simulink model "synchronverter_simulation"  (R2023a)
settings: Solver=ode23tb  StartTime=0.0  StopTime=9  FixedStep=1e-5  MaxStep=0.2e-3  RelTol=1e-3
model workspace (MAT data in the model file):
  Dp = 0.2026
  Dq = 117.88
  Ki = 9
  Kp = 1
  L = 0.0002
  Lg = 0.00015
  Ls = 0.00045
  Pset = 80
  Qset = 60
  R = 0.05
  Rg = 0.045
  Rs = 0.135
  Vdclink = 42
  Vlgrms = 380
  Vnpeak = 16.9667989517
  Wn = 314.159265359
  Ws = 94247.7796077
  fg = 50
  fs = 15000
  tf = 0.002
  tv = 0.02
libraries: simulink_extras x5, spsThreePhaseVIMeasurementLib x5, spsThreePhaseBreakerLib x4, spsPower3phInstantaneousLib x4, cstblocks x3, spsGroundLib x3, spsThreePhaseParallelRLCLoadLib x2, spsThreePhaseSeriesRLCBranchLib x2, spsDCVoltageSourceLib x2, spsThreePhaseProgrammableVoltageSourceLib x1, spsThreePhaseParallelRLCBranchLib x1, slpidlib x1
settings Model: Creator=Hi  LastModifiedBy=Aminsystem
settings SolverCC: AlgebraicLoopSolver=TrustRegion
settings DataIOCC: ReturnWorkspaceOutputs=off
settings DebuggingCC: AlgebraicLoopMsg=none  ArithmeticOperatorsInVariantConditions=warning
settings ModelReferenceCC: EnableRefExpFcnMdlSchedulingChecks=on
settings SFSimCC: SimUseLocalCustomCode=off  CustomCodeUndefinedFunction=UseInterfaceOnly
settings RTWCC: RTWUseLocalCustomCode=off
settings ConfigComp: DVTestSuiteOptimization=CombinedObjectives (Nonlinear Extended)

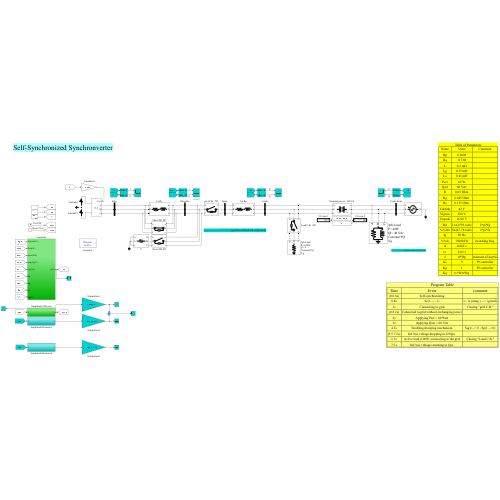
[thumbnail: Simulink's stored preview of the top-level diagram]
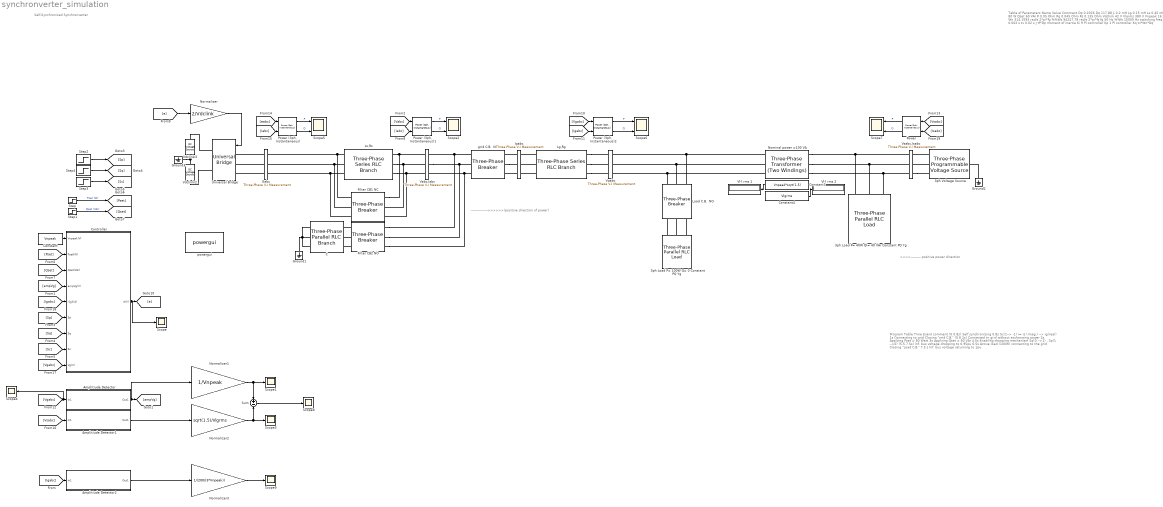
== system synchronverter_simulation ==
  note: <<<<---------- positive power direction
  note: ----------------->>>>>>(positive direction of power)
  note: Table of Parameters
      | Name
      | Value
      | Comment
      |
      | Dp
      | 0.2026
      |
      | Dq
      | 117.88
      |
      | L
      | 0.2 mH
      |
      | Lg
      | 0.15 mH
      |
      | Ls
      | 0.45 mH
      |
      | Pset
      | 80 W
      |
      | Qset
      | 60 VAr
      |
      | R
      | 0.05 Ohm
      |
      | Rg
      | 0.045 Ohm
      |
      | Rs
      | 0.135 Ohm
      |
      | Vdclink
      | 42 V
      |
      | Vlgrms
      | 380 V
      |
      | Vnpeak
      | 16.96 V
      |
      | Wn
      | 314.1593 rad/s
      | 2*pi*fg
      |
      | %%Ws
      | 94247.78 rad/s
      | 2*pi*fs
      |
      | fg
      | 50 Hz
      |
      | %%fs
      | 15000 Hz
      | switching freq.
      |
      | tf
      | 0.002 s
      |
      | tv
      | 0.02 s
      |
      | J
      | tf*Dp
      | moment of inertia
      |
      | Ki
      | 9
      | PI controller
      |
      | Kp
      | 1
      | PI controller
      |
      | Kq
      | tv*Wn*Dq
  note: Program Table
      | Time
      | Event
      | comment
      |
      | (0 0.8s)
      | Self synchronizing
      |
      | 0.8s
      | Sc(1--> -1)
      | i= is (imag.) --> ig(real)
      |
      | 1s
      | Connecting to grid
      | Closing "grid C.B."
      |
      | (0.8 2s)
      | Connected to grid without exchanging power
      |
      | 2s
      | Applying Pset = 80 Watt
      |
      | 3s
      | Applying Qset = 60 VAr
      |
      | 4.5s
      | Enabling drooping mechanism
      | Sq(0 -->1) , Sp(1 -->0)
      |
      | (5.5 7.5s)
      | Inf. bus voltage dropping to 0.95pu
      |
      | 6.5s
      | Active load (100W) connecting to the grid
      | Closing "Load C.B."
      |
      | 7.5 s
      | Inf. bus voltage returning to 1pu
  note: Self-Synchronized Synchronverter
  3ph Voltage Source : spsThreePhaseProgrammableVoltageSourceLib/Three-Phase Programmable Voltage Source  PositiveSequence=[Vlgrms 0 fg]  VariationEntity=Amplitude  VariationType=Table of time-amplitude pairs  VariationTypeAlt=Step  VariationStep=0.5  VariationRate=10  VariationMagnitude=0.3  VariationFrequency=2  VariationTiming=[1 2]  VariationPhaseA=off  Amplitudes=[1 0.95 1]  TimeValues=[0 5.5 7.5]  HarmonicGeneration=off  HarmonicA=[3 0.2 -25 0]  HarmonicB=[2 0.15 35 2]  Timing="[0.05  3]"  BusType=swing  Pref=0  Qref=0  Qmin=-inf  Qmax=inf
  3ph Load P= 100W Q= 0 Constant PQ Yg : spsThreePhaseParallelRLCLoadLib/Three-Phase Parallel RLC Load  LConnTagsString=A|B|C  Configuration=Y (grounded)  NominalVoltage=Vnpeak*sqrt(1.5)  Vabc=[1e3 1e3 1e3]  Vabcp=[1e3 1e3 1e3]  NominalFrequency=fg  UnbalancedPower=off  ActivePower=100  InductivePower=0  CapacitivePower=0  Pabc=[10e3 9e3 11e3]  QLabc=[100 90 110]  QCabc=[100 90 110]  Pabcp=[10e3 9e3 11e3]  QLabcp=[100 90 110]  QCabcp=[100 90 110]  Measurements=None  LoadType=constant PQ
  3ph Load P= 40W Ql= 40 VAr Constant PQ Yg : spsThreePhaseParallelRLCLoadLib/Three-Phase Parallel RLC Load  LConnTagsString=A|B|C  Configuration=Y (grounded)  NominalVoltage=Vlgrms  Vabc=[1e3 1e3 1e3]  Vabcp=[1e3 1e3 1e3]  NominalFrequency=fg  UnbalancedPower=off  ActivePower=40  InductivePower=40  CapacitivePower=0  Pabc=[10e3 9e3 11e3]  QLabc=[100 90 110]  QCabc=[100 90 110]  Pabcp=[10e3 9e3 11e3]  QLabcp=[100 90 110]  QCabcp=[100 90 110]  Measurements=None  LoadType=constant PQ
  Amplitiude Detector : Subsystem
  Amplitiude Detector1 : Subsystem
  Amplitiude Detector2 : Subsystem
  C : spsThreePhaseParallelRLCBranchLib/Three-Phase Parallel RLC Branch  LConnTagsString=A|B|C  RConnTagsString=A|B|C  BranchType=C  Resistance=inf  Inductance=1e3  Capacitance=1/(L*Wn*Ws)*1+(22e-6)*0  Measurements=None
  Constant : Constant  Value=Vnpeak
  Constant3 : Constant  Value=Vnpeak*sqrt(1.5)
  Constant4 : Constant  Value=Vlgrms
  Controller : Subsystem
  Eabc : spsThreePhaseVIMeasurementLib/Three-Phase V-I Measurement  VoltageMeasurement=phase-to-ground  SetLabelV=on  LabelV=eabc  Vpu=off  VpuLL=off  CurrentMeasurement=no  SetLabelI=on  LabelI=Iabc  Ipu=off  Pbase=100e6  Vbase=500e3  OutputType=Complex  PhasorSimulation=off  PSBequivalent=0
  Filter CB1 NC : spsThreePhaseBreakerLib/Three-Phase Breaker  InitialState=closed  SwitchA=on  SwitchB=on  SwitchC=on  SwitchTimes=[500]  External=off  BreakerResistance=0.01  SnubberResistance=1e7  SnubberCapacitance=inf  Measurements=None
  Filter CB2 NO : spsThreePhaseBreakerLib/Three-Phase Breaker  InitialState=open  SwitchA=on  SwitchB=on  SwitchC=on  SwitchTimes=[500]  External=off  BreakerResistance=0.01  SnubberResistance=1e7  SnubberCapacitance=inf  Measurements=None
  Ground1 : spsGroundLib/Ground  LConnTagsString=a
  Ground2 : spsGroundLib/Ground  LConnTagsString=a
  Ground3 : spsGroundLib/Ground  LConnTagsString=a
  Igabc : spsThreePhaseVIMeasurementLib/Three-Phase V-I Measurement  VoltageMeasurement=no  SetLabelV=off  LabelV=Vg3  Vpu=off  VpuLL=off  CurrentMeasurement=yes  SetLabelI=on  LabelI=Igabc  Ipu=off  Pbase=100e6  Vbase=500e3  OutputType=Complex  PhasorSimulation=off  PSBequivalent=0
  Lg,Rg : spsThreePhaseSeriesRLCBranchLib/Three-Phase Series RLC Branch  LConnTagsString=A|B|C  RConnTagsString=A|B|C  BranchType=RL  Resistance=Rg  Inductance=Lg  Capacitance=1e-6  Measurements=None
  Load C.B.  NO : spsThreePhaseBreakerLib/Three-Phase Breaker  InitialState=open  SwitchA=on  SwitchB=on  SwitchC=on  SwitchTimes=[6.5]  External=off  BreakerResistance=0.01  SnubberResistance=1e6  SnubberCapacitance=inf  Measurements=Breaker voltages
  Ls,Rs : spsThreePhaseSeriesRLCBranchLib/Three-Phase Series RLC Branch  LConnTagsString=A|B|C  RConnTagsString=A|B|C  BranchType=RL  Resistance=Rs  Inductance=Ls  Capacitance=1e-6  Measurements=None
  Nominal power =100 VA : spsThreePhaseTransformerTwoWindingsLib/Three-Phase Transformer (Two Windings)  Winding1Connection=Yg  Winding2Connection=Yg  CoreType=Three single-phase transformers  SetSaturation=off  Hysteresis=off  DataFile='hysteresis'  SetInitialFlux=off  Measurements=None  UNITS=pu  NominalPower=[ 100 , fg ]  Winding1=[ Vnpeak*sqrt(1.5) , 0.002 , 0.08 ]  Winding2=[Vlgrms , 0.002 , 0.08 ]  Rm=500  Lm=500  L0=0.5  Saturation=[ 0,0 ; 0.0024,1.2 ; 1.0,1.52 ]  InitialFluxes=[ 0.8 , -0.8 , 0.7 ]  BreakLoop=off  DiscreteSolver=Trapezoidal iterative  DataType=off  TransfoNumber=1
  Normalizer : Gain  Gain=2/Vdclink
  Normalizer1 : Gain  Gain=1/Vnpeak
  Normalizer2 : Gain  Gain=sqrt(1.5)/Vlgrms
  Normalizer3 : Gain  Gain=1/(200/(3*Vnpeak))
  Power : spsPower3phInstantaneousLib/Power (3ph, Instantaneous)
  "Power (3ph, Instantaneous)" : spsPower3phInstantaneousLib/Power (3ph, Instantaneous)
  "Power (3ph, Instantaneous)1" : spsPower3phInstantaneousLib/Power (3ph, Instantaneous)
  "Power (3ph, Instantaneous)2" : spsPower3phInstantaneousLib/Power (3ph, Instantaneous)
  Scope{,1,3..4,8..9} (6 alike) : Scope
  Scope{2,5..7} (4 alike) : Scope  NumInputPorts=2
  Step : Step  Time=2  After=Pset  SampleTime=0
  Step1 : Step  Time=3  After=Qset  SampleTime=0
  Step2 : Step  Time=4.5  Before=1  After=-1  SampleTime=0
  Step3 : Step  Time=0.8  Before=1  After=-1  SampleTime=0
  Step4 : Step  Time=4.5  SampleTime=0
  Sum : Sum  Inputs=+|-
  Universal Bridge : spsUniversalBridgeLib/Universal Bridge  Arms=3  SnubberResistance=inf  SnubberCapacitance=inf  Device=Average-model based VSC  Ron=1e-3  Lon=0  ForwardVoltages="[  0  0  ]"  ForwardVoltage=0  GTOparameters=[ 10e-6 , 20e-6 ]  IGBTparameters=[ 1e-6 , 2e-6 ]  Measurements=None  Measurements_2=None  converterType=Rectifier
  Vabc,Iabc : spsThreePhaseVIMeasurementLib/Three-Phase V-I Measurement  VoltageMeasurement=phase-to-ground  SetLabelV=on  LabelV=Vabc  Vpu=off  VpuLL=off  CurrentMeasurement=yes  SetLabelI=on  LabelI=Iabc  Ipu=off  Pbase=100e6  Vbase=500e3  OutputType=Complex  PhasorSimulation=off  PSBequivalent=0
  Vdclink/2 : spsDCVoltageSourceLib/DC Voltage Source  Amplitude=Vdclink/2  Measurements=None
  Vdclink/2. : spsDCVoltageSourceLib/DC Voltage Source  Amplitude=Vdclink/2  Measurements=None
  Vgabc : spsThreePhaseVIMeasurementLib/Three-Phase V-I Measurement  VoltageMeasurement=phase-to-ground  SetLabelV=on  LabelV=Vgabc  Vpu=off  VpuLL=off  CurrentMeasurement=no  SetLabelI=off  LabelI=Ig3  Ipu=off  Pbase=100  Vbase=Vnpeak*sqrt(1.5)  OutputType=Complex  PhasorSimulation=off  PSBequivalent=0
  Vl-l rms 1 : Display
  Vl-l rms 2 : Display
  Vsabc,Isabc : spsThreePhaseVIMeasurementLib/Three-Phase V-I Measurement  VoltageMeasurement=phase-to-ground  SetLabelV=on  LabelV=Vsabc  Vpu=off  VpuLL=off  CurrentMeasurement=yes  SetLabelI=on  LabelI=Isabc  Ipu=off  Pbase=100e6  Vbase=500e3  OutputType=Complex  PhasorSimulation=off  PSBequivalent=0
  grid C.B.  NO : spsThreePhaseBreakerLib/Three-Phase Breaker  InitialState=open  SwitchA=on  SwitchB=on  SwitchC=on  SwitchTimes=[1]  External=off  BreakerResistance=0.01  SnubberResistance=1e6  SnubberCapacitance=inf  Measurements=Breaker voltages
  powergui : sps_lib/powergui  Priority=1  SimulationMode=Discrete  SampleTime=5e-5  frequency=Ws/(2*pi)  Iterations=50  frequencyindice=0  Pbase=100  ErrMax=1e-2  UnitsV=V  UnitsW=W  buscounter=0  FunctionMessages=off  echomessages=off  EnableUseOfTLC=off  CurrentSourceSwitches=off  DisableSnubberDevices=off  DisableRonSwitches=off  DisableVfSwitches=off  DisplayEquations=off  AutomaticDiscreteSolvers=off  SolverType=Tustin/Backward Euler (TBE)  Interpol=off  ExternalGateDelay=off  methode=off  Ts=100  x0status=blocks  SPID=off  SwTol=0  HookPort=off  NonlinearTolerance=1e-4  nMaxIteration=100  ContinueOnMaxIteration=off  RestoreLinks=warning  ResistiveCurrentMeasurement=off  Frange=[0:2:500]  Ylog=off  Xlog=on  ShowGrid=off  save=off  variable=ZData  structure=0  ZoomFFT=off  StartTime=0.0  cycles=1  DisplayStyle=1  fundamental=60  FreqAxis=off  MaxFrequency=1000  frequencyindicesteady=1  RmsSteady=1  display=off
  wires:
  [ampVg] -> Controller/4(ampVg(V))
  [Sc] -> Controller/8(Sc)
  [Sq] -> Controller/7(Sq)
  [Sp] -> Controller/6(Sp)
  [Pset] -> Controller/2(Pset(W))
  [Qset] -> Controller/3(Qset(VAr))
  Step3/1 -> [Sc]
  Step4/1 -> [Sq]
  Step2/1 -> [Sp]
  Normalizer/1 -> Universal Bridge/1
  Controller/1(e(V)) -> Scope/1, [e]
  [e] -> Normalizer/1
  [Vgabc] -> Scope4/1, Amplitiude Detector/1(In1)
  Amplitiude Detector/1(Out1) -> [ampVg], Normalizer1/1
  Step1/1 -> [Qset]  "Qset (VAr)"
  Step/1 -> [Pset]  "Pset (W)"
  Constant/1 -> Controller/1(Vnpeak(V))
  [Igabc] -> Controller/5("i{g}(A)")
  [Vgabc] -> Controller/9(Vg(V))
  [eabc] -> "Power (3ph, Instantaneous)"/1
  [Iabc] -> "Power (3ph, Instantaneous)"/2
  "Power (3ph, Instantaneous)"/1 -> Scope5/1  "P"
  "Power (3ph, Instantaneous)"/2 -> Scope5/2  "Q"
  Constant3/1 -> Vl-l rms 1/1
  Constant4/1 -> Vl-l rms 2/1
  "Power (3ph, Instantaneous)1"/2 -> Scope2/2  "Q"
  [Vabc] -> "Power (3ph, Instantaneous)1"/1
  "Power (3ph, Instantaneous)1"/1 -> Scope2/1  "P"
  [Iabc] -> "Power (3ph, Instantaneous)1"/2
  "Power (3ph, Instantaneous)2"/1 -> Scope6/1  "P"
  [Igabc] -> "Power (3ph, Instantaneous)2"/2
  "Power (3ph, Instantaneous)2"/2 -> Scope6/2  "Q"
  [Vgabc] -> "Power (3ph, Instantaneous)2"/1
  Power/1 -> Scope7/1  "P"
  Power/2 -> Scope7/2  "Q"
  [Vsabc] -> Power/1
  [Isabc] -> Power/2
  Normalizer1/1 -> Scope1/1, Sum/1
  [Vsabc] -> Amplitiude Detector1/1(In1)
  Amplitiude Detector1/1(Out1) -> Normalizer2/1
  Normalizer2/1 -> Scope3/1, Sum/2
  Sum/1 -> Scope8/1
  [Igabc] -> Amplitiude Detector2/1(In1)
  Amplitiude Detector2/1(Out1) -> Normalizer3/1
  Normalizer3/1 -> Scope9/1
  connections:
  Universal Bridge/RConn1 -- Vdclink/2/RConn1
  Vdclink/2./LConn1 -- Universal Bridge/RConn2
  Ground2/LConn1 -- 3ph Voltage Source/LConn1
  grid C.B.  NO/LConn1 -- Vabc,Iabc/RConn1 -- Filter CB2 NO/RConn1
  Vabc,Iabc/RConn2 -- Filter CB2 NO/RConn2 -- grid C.B.  NO/LConn2
  grid C.B.  NO/LConn3 -- Vabc,Iabc/RConn3 -- Filter CB2 NO/RConn3
  Vdclink/2./RConn1 -- Ground3/LConn1 -- Vdclink/2/LConn1
  Igabc/LConn1 -- grid C.B.  NO/RConn1
  Lg,Rg/LConn2 -- Igabc/RConn2
  Lg,Rg/LConn3 -- Igabc/RConn3
  Lg,Rg/LConn1 -- Igabc/RConn1
  Eabc/LConn1 -- Universal Bridge/LConn1
  Eabc/LConn2 -- Universal Bridge/LConn2
  Eabc/LConn3 -- Universal Bridge/LConn3
  grid C.B.  NO/RConn2 -- Igabc/LConn2
  Igabc/LConn3 -- grid C.B.  NO/RConn3
  C/RConn3 -- C/RConn1 -- Ground1/LConn1 -- C/RConn2
  Lg,Rg/RConn1 -- Vgabc/LConn1
  Lg,Rg/RConn2 -- Vgabc/LConn2
  Lg,Rg/RConn3 -- Vgabc/LConn3
  Nominal power =100 VA/LConn1 -- Load C.B.  NO/LConn1 -- Vgabc/RConn1
  Nominal power =100 VA/LConn2 -- Load C.B.  NO/LConn2 -- Vgabc/RConn2
  Nominal power =100 VA/LConn3 -- Load C.B.  NO/LConn3 -- Vgabc/RConn3
  Nominal power =100 VA/RConn1 -- Vsabc,Isabc/RConn1 -- 3ph Load P= 40W Ql= 40 VAr Constant PQ Yg/LConn1
  Nominal power =100 VA/RConn2 -- Vsabc,Isabc/RConn2 -- 3ph Load P= 40W Ql= 40 VAr Constant PQ Yg/LConn2
  Nominal power =100 VA/RConn3 -- Vsabc,Isabc/RConn3 -- 3ph Load P= 40W Ql= 40 VAr Constant PQ Yg/LConn3
  Filter CB2 NO/LConn1 -- C/LConn1
  Filter CB2 NO/LConn2 -- C/LConn2
  Filter CB2 NO/LConn3 -- C/LConn3
  Filter CB1 NC/RConn1 -- Vabc,Iabc/LConn1 -- Ls,Rs/RConn1
  Vabc,Iabc/LConn2 -- Ls,Rs/RConn2 -- Filter CB1 NC/RConn2
  Vabc,Iabc/LConn3 -- Ls,Rs/RConn3 -- Filter CB1 NC/RConn3
  Ls,Rs/LConn1 -- Filter CB1 NC/LConn1 -- Eabc/RConn1
  Ls,Rs/LConn2 -- Filter CB1 NC/LConn2 -- Eabc/RConn2
  Ls,Rs/LConn3 -- Filter CB1 NC/LConn3 -- Eabc/RConn3
  3ph Voltage Source/RConn1 -- Vsabc,Isabc/LConn1
  3ph Voltage Source/RConn2 -- Vsabc,Isabc/LConn2
  Vsabc,Isabc/LConn3 -- 3ph Voltage Source/RConn3
  3ph Load P= 100W Q= 0 Constant PQ Yg/LConn1 -- Load C.B.  NO/RConn3
  3ph Load P= 100W Q= 0 Constant PQ Yg/LConn2 -- Load C.B.  NO/RConn2
  3ph Load P= 100W Q= 0 Constant PQ Yg/LConn3 -- Load C.B.  NO/RConn1

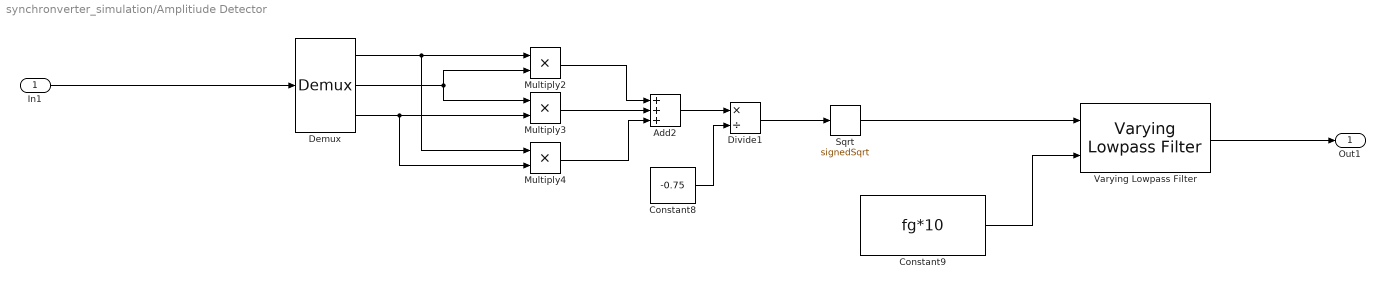
== system synchronverter_simulation/Amplitiude Detector ==
  In1 : Inport
  Add2 : Sum  Inputs=3
  Constant8 : Constant  Value=-0.75
  Constant9 : Constant  Value=fg*10
  Demux : Demux  Outputs=3
      settings: DisplayOption=none
  Divide1 : Product  Inputs=*/
  Multiply2 : Product
  Multiply3 : Product
  Multiply4 : Product
  Sqrt : Sqrt  Operator=signedSqrt
  Varying Lowpass Filter : cstblocks/Linear Parameter Varying/Varying Lowpass Filter  N=1
  Out1 : Outport  VectorParamsAs1DForOutWhenUnconnected=off
  wires:
  Demux/2 -> Multiply2/2, Multiply3/1
  Add2/1 -> Divide1/1
  Sqrt/1 -> Varying Lowpass Filter/1
  Constant8/1 -> Divide1/2
  Demux/1 -> Multiply4/1, Multiply2/1
  Constant9/1 -> Varying Lowpass Filter/2
  Varying Lowpass Filter/1 -> Out1/1
  In1/1 -> Demux/1
  Demux/3 -> Multiply4/2, Multiply3/2
  Multiply2/1 -> Add2/1
  Multiply3/1 -> Add2/2
  Divide1/1 -> Sqrt/1
  Multiply4/1 -> Add2/3

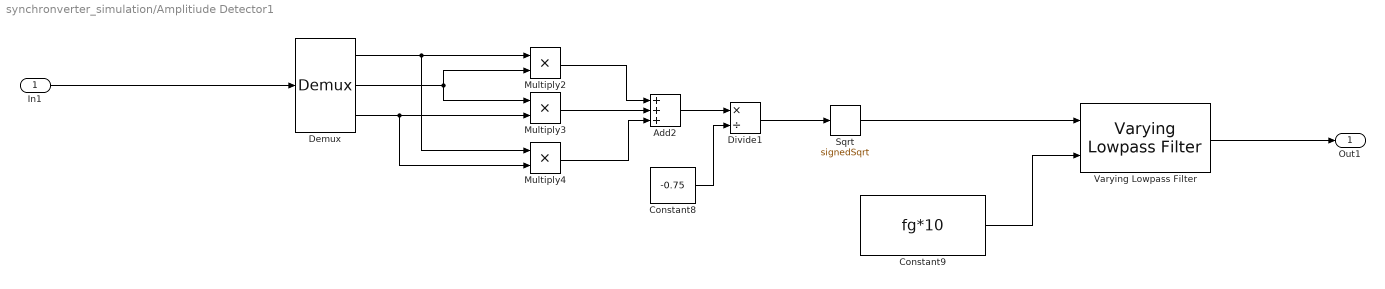
== system synchronverter_simulation/Amplitiude Detector1 ==
  In1 : Inport
  Add2 : Sum  Inputs=3
  Constant8 : Constant  Value=-0.75
  Constant9 : Constant  Value=fg*10
  Demux : Demux  Outputs=3
      settings: DisplayOption=none
  Divide1 : Product  Inputs=*/
  Multiply2 : Product
  Multiply3 : Product
  Multiply4 : Product
  Sqrt : Sqrt  Operator=signedSqrt
  Varying Lowpass Filter : cstblocks/Linear Parameter Varying/Varying Lowpass Filter  N=1
  Out1 : Outport  VectorParamsAs1DForOutWhenUnconnected=off
  wires:
  Demux/2 -> Multiply2/2, Multiply3/1
  Add2/1 -> Divide1/1
  Sqrt/1 -> Varying Lowpass Filter/1
  Constant8/1 -> Divide1/2
  Demux/1 -> Multiply4/1, Multiply2/1
  Constant9/1 -> Varying Lowpass Filter/2
  Varying Lowpass Filter/1 -> Out1/1
  In1/1 -> Demux/1
  Demux/3 -> Multiply4/2, Multiply3/2
  Multiply2/1 -> Add2/1
  Multiply3/1 -> Add2/2
  Divide1/1 -> Sqrt/1
  Multiply4/1 -> Add2/3

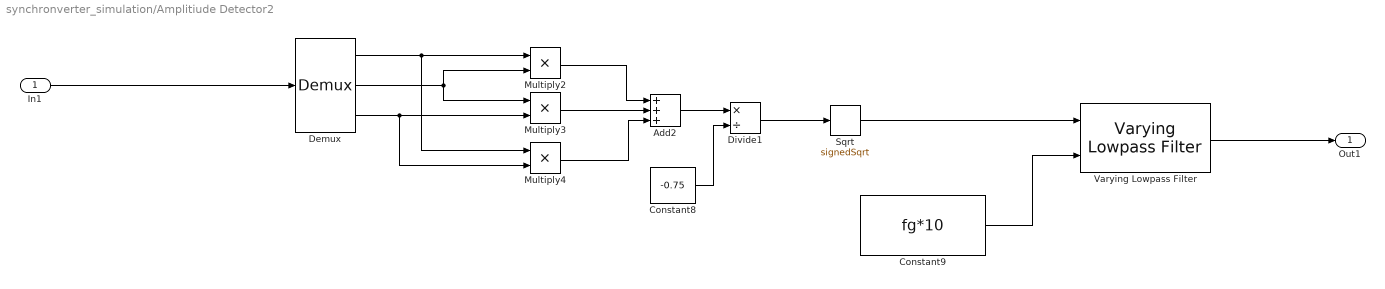
== system synchronverter_simulation/Amplitiude Detector2 ==
  In1 : Inport
  Add2 : Sum  Inputs=3
  Constant8 : Constant  Value=-0.75
  Constant9 : Constant  Value=fg*10
  Demux : Demux  Outputs=3
      settings: DisplayOption=none
  Divide1 : Product  Inputs=*/
  Multiply2 : Product
  Multiply3 : Product
  Multiply4 : Product
  Sqrt : Sqrt  Operator=signedSqrt
  Varying Lowpass Filter : cstblocks/Linear Parameter Varying/Varying Lowpass Filter  N=1
  Out1 : Outport  VectorParamsAs1DForOutWhenUnconnected=off
  wires:
  Demux/2 -> Multiply2/2, Multiply3/1
  Add2/1 -> Divide1/1
  Sqrt/1 -> Varying Lowpass Filter/1
  Constant8/1 -> Divide1/2
  Demux/1 -> Multiply4/1, Multiply2/1
  Constant9/1 -> Varying Lowpass Filter/2
  Varying Lowpass Filter/1 -> Out1/1
  In1/1 -> Demux/1
  Demux/3 -> Multiply4/2, Multiply3/2
  Multiply2/1 -> Add2/1
  Multiply3/1 -> Add2/2
  Divide1/1 -> Sqrt/1
  Multiply4/1 -> Add2/3

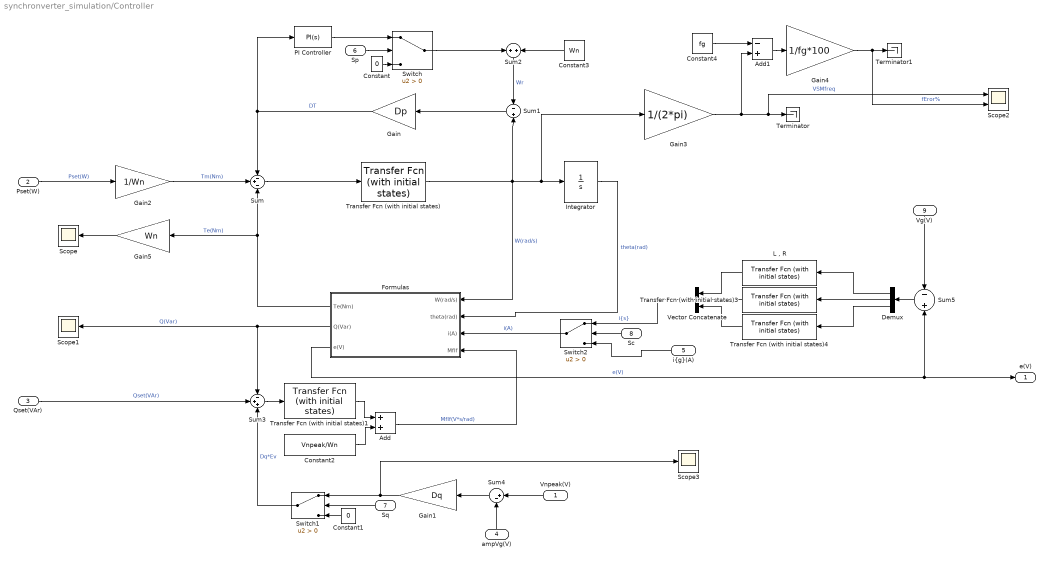
== system synchronverter_simulation/Controller ==
  Vnpeak(V) : Inport  Unit=V
  Pset(W) : Inport  Port=2  Unit=W
  Qset(VAr) : Inport  Port=3  Unit=W
  ampVg(V) : Inport  Port=4  Unit=V
  "i{g}(A)" : Inport  Port=5  Unit=A
  Sp : Inport  Port=6
  Sq : Inport  Port=7
  Sc : Inport  Port=8
  Vg(V) : Inport  Port=9  Unit=V
  Add : Sum
  Add1 : Sum  Inputs=-+
  Constant : Constant  Value=0
  Constant1 : Constant  Value=0
  Constant2 : Constant  Value=Vnpeak/Wn
  Constant3 : Constant  Value=Wn
  Constant4 : Constant  Value=fg
  Demux : Demux  Outputs=3
  Formulas : Subsystem
  Gain : Gain  Gain=Dp
  Gain1 : Gain  Gain=Dq
  Gain2 : Gain  Gain=1/Wn
  Gain3 : Gain  Gain=1/(2*pi)
  Gain4 : Gain  Gain=1/fg*100
  Gain5 : Gain  Gain=Wn
  Integrator : Integrator  WrapState=on  WrappedStateUpperValue=2*pi  WrappedStateLowerValue=0  ZeroCross=off
  "L , R" : simulink_extras/Additional Linear/Transfer Fcn (with initial states)  N=[1]  D=[L R]  X0=0
  PI Controller : slpidlib/PID Controller  Controller=PI  Form=Parallel  TimeDomain=Continuous-time  UseExternalTs=off  SampleTime=-1  IntegratorMethod=Forward Euler  FilterMethod=Forward Euler  ControllerParametersSource=internal  P=Kp  I=Ki  UseKiTs=off  D=0  N=100  UseFilter=on  TunerSelectOption=Transfer Function Based (PID Tuner App)  ZeroCross=off  InitialConditionSource=internal  InitialConditionForIntegrator=0  InitialConditionForFilter=0  DifferentiatorICPrevScaledInput=0  ExternalReset=none  TrackingMode=off  Kt=1  LimitOutput=off  SatLimitsSource=internal  UpperSaturationLimit=inf  LowerSaturationLimit=-inf  LinearizeAsGain=on  AntiWindupMode=none  Kb=1  LimitIntegrator=off  UpperIntegratorSaturationLimit=inf  LowerIntegratorSaturationLimit=-inf  POutMin=[]  POutMax=[]  IOutMin=[]  IOutMax=[]  DOutMin=[]  DOutMax=[]  NOutMin=[]  NOutMax=[]  SumOutMin=[]  SumOutMax=[]  SaturationOutMin=[]  SaturationOutMax=[]  PParamMin=[]  PParamMax=[]  IParamMin=[]  IParamMax=[]  DParamMin=[]  DParamMax=[]  NParamMin=[]  NParamMax=[]  KbParamMin=[]  KbParamMax=[]  KtParamMin=[]  KtParamMax=[]  KbOutMin=[]  KbOutMax=[]  KtOutMin=[]  KtOutMax=[]  IntegratorOutMin=[]  IntegratorOutMax=[]  FilterOutMin=[]  FilterOutMax=[]  SumI1OutMin=[]  SumI1OutMax=[]  SumI2OutMin=[]  SumI2OutMax=[]  SumI3OutMin=[]  SumI3OutMax=[]  SumI4OutMin=[]  SumI4OutMax=[]  SumDOutMin=[]  SumDOutMax=[]  DifferentiatorOutMin=[]  DifferentiatorOutMax=[]  FilterDiffOutCoefMin=[]  FilterDiffOutCoefMax=[]  ReciprocalOutMin=[]  ReciprocalOutMax=[]  SumDenOutMin=[]  SumDenOutMax=[]  SumNumOutMin=[]  SumNumOutMax=[]  DivideOutMin=[]  DivideOutMax=[]  UdiffTsProdOutMin=[]  UdiffTsProdOutMax=[]  NTsProdOutMin=[]  NTsProdOutMax=[]  UintegralTsProdOutMin=[]  UintegralTsProdOutMax=[]  UngainTsProdOutMin=[]  UngainTsProdOutMax=[]  ClampingZeroOutDataTypeStr=Inherit: Inherit via back propagation  ClampingZeroOutMin=[]  ClampingZeroOutMax=[]  FilterDenConstantOutDataTypeStr=Inherit: Inherit via back propagation  FilterDenConstantOutMin=[]  FilterDenConstantOutMax=[]  PCopyOutDataTypeStr=Inherit: Inherit via back propagation  PCopyOutMin=[]  PCopyOutMax=[]  NCopyOutDataTypeStr=Inherit: Inherit via back propagation  NCopyOutMin=[]  NCopyOutMax=[]  IntegratorContinuousStateAttributes=''  IntegratorStateMustResolveToSignalObject=off  IntegratorRTWStateStorageClass=Auto  FilterContinuousStateAttributes=''  FilterStateMustResolveToSignalObject=off  FilterRTWStateStorageClass=Auto  ParallelPVariant=InternalParameters  IdealPVariant=Disabled  IVariant=InternalParameters  DVariant=Disabled  IntegratorVariant=Continuous  SatVariant=Disabled  AWVariant=Passthrough  PCopyVariant=Disabled  TRVariant=Disabled  FdbkBlocksVariant=Forward  IdealPFdbkVariant=Disabled  SatFdbkVariant=Disabled  DerivativeFilterVariant=Disabled  NVariant=Disabled  NCopyVariant=Disabled_SignalSpec  FilterICVariant=Disabled  IntegratorICVariant=InternalICs  ExternalResetVariant=Disabled  TRSumVariant=Passthrough  SumFdbkVariant=Disabled  SumVariant=Sum_PI  TsampFilterVariant=InternalTs  TsampNgainVariant=Passthrough  TsampIntegralVariant=Disabled_SignalSpec  ExternalSaturationOutDataTypeStr=Inherit: Same as second input
  Scope : Scope
  Scope1 : Scope
  Scope2 : Scope  NumInputPorts=2
  Scope3 : Scope
  Sum : Sum  Inputs=-+-
  Sum1 : Sum  Inputs=-+
  Sum2 : Sum  Inputs=+|+
  Sum3 : Sum  Inputs=-++
  Sum4 : Sum  Inputs=|+-
  Sum5 : Sum  Inputs=-+
  Switch : Switch  Criteria=u2 > Threshold  SaturateOnIntegerOverflow=off  InputSameDT=off
  Switch1 : Switch  Criteria=u2 > Threshold  SaturateOnIntegerOverflow=off  InputSameDT=off
  Switch2 : Switch  Criteria=u2 > Threshold  SaturateOnIntegerOverflow=off  InputSameDT=off
  Terminator : Terminator
  Terminator1 : Terminator
  Transfer Fcn (with initial states) : simulink_extras/Additional Linear/Transfer Fcn (with initial states)  N=[1]  D=[(tf*Dp) 0]  X0=0
  Transfer Fcn (with initial states)1 : simulink_extras/Additional Linear/Transfer Fcn (with initial states)  N=[1]  D=[tv*Wn*Dq 0]  X0=0
  Transfer Fcn (with initial states)3 : simulink_extras/Additional Linear/Transfer Fcn (with initial states)  N=[1]  D=[L R]  X0=0
  Transfer Fcn (with initial states)4 : simulink_extras/Additional Linear/Transfer Fcn (with initial states)  N=[1]  D=[L R]  X0=0
  Vector Concatenate : Concatenate  NumInputs=3
  e(V) : Outport  Unit=V  VectorParamsAs1DForOutWhenUnconnected=off
  wires:
  Pset(W)/1 -> Gain2/1  "Pset(W)"
  Gain2/1 -> Sum/2  "Tm(Nm)"
  Gain/1 -> PI Controller/1, Sum/1  "DT"
  Sum1/1 -> Gain/1
  PI Controller/1 -> Switch/1
  Sp/1 -> Switch/2
  Constant/1 -> Switch/3
  Switch/1 -> Sum2/1
  Sum2/1 -> Sum1/1  "Wr"
  Sum/1 -> Transfer Fcn (with initial states)/1
  Transfer Fcn (with initial states)/1 -> Integrator/1, Gain3/1, Sum1/2, Formulas/1(W(rad/s))  "W(rad/s)"
  Formulas/1(Te(Nm)) -> Gain5/1, Sum/3  "Te(Nm)"
  Qset(VAr)/1 -> Sum3/2  "Qset(VAr)"
  Formulas/2(Q(Var)) -> Sum3/1, Scope1/1  "Q(Var)"
  Sum3/1 -> Transfer Fcn (with initial states)1/1
  Transfer Fcn (with initial states)1/1 -> Add/1
  Sq/1 -> Switch1/2
  Constant1/1 -> Switch1/3
  Switch1/1 -> Sum3/3  "Dq*Ev"
  Gain1/1 -> Scope3/1, Switch1/1
  Sum4/1 -> Gain1/1
  ampVg(V)/1 -> Sum4/2
  Vnpeak(V)/1 -> Sum4/1
  Sc/1 -> Switch2/2
  "i{g}(A)"/1 -> Switch2/3
  Switch2/1 -> Formulas/3(i(A))  "i(A)"
  Integrator/1 -> Formulas/2(theta(rad))  "theta(rad)"
  Constant3/1 -> Sum2/2
  Vg(V)/1 -> Sum5/1
  Formulas/3(e(V)) -> Sum5/2, e(V)/1  "e(V)"
  Gain3/1 -> Add1/2, Scope2/1, Terminator/1  "VSMfreq"
  Add/1 -> Formulas/4(MfIf)  "MfIf(V*s/rad)"
  Sum5/1 -> Demux/1
  Demux/1 -> "L , R"/1
  Demux/2 -> Transfer Fcn (with initial states)3/1
  Demux/3 -> Transfer Fcn (with initial states)4/1
  Transfer Fcn (with initial states)3/1 -> Vector Concatenate/2
  Vector Concatenate/1 -> Switch2/1  "i{s}"
  "L , R"/1 -> Vector Concatenate/1
  Transfer Fcn (with initial states)4/1 -> Vector Concatenate/3
  Gain4/1 -> Scope2/2, Terminator1/1  "fEror%"
  Add1/1 -> Gain4/1
  Constant4/1 -> Add1/1
  Constant2/1 -> Add/2
  Gain5/1 -> Scope/1

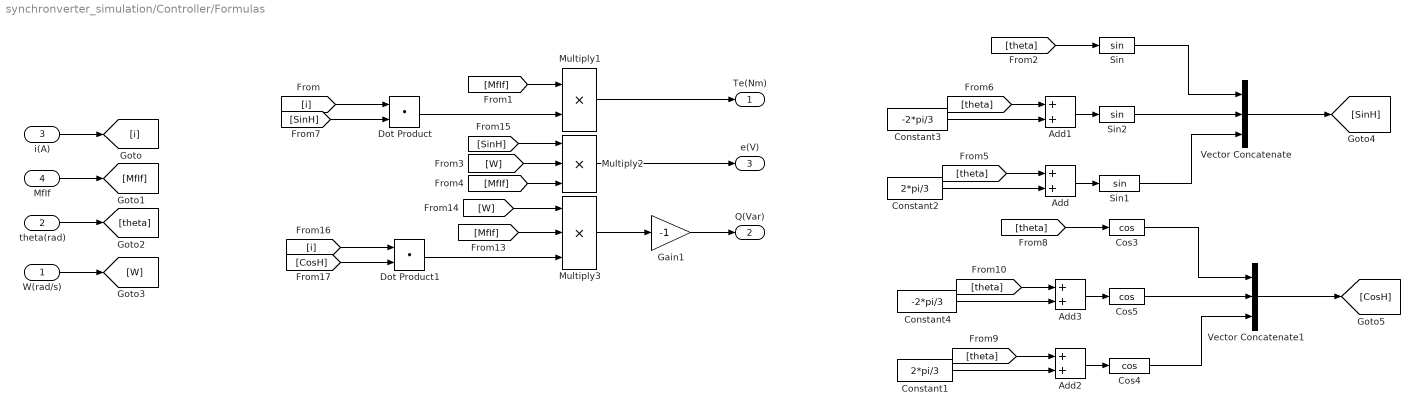
== system synchronverter_simulation/Controller/Formulas ==
  W(rad/s) : Inport  Unit=rad/s
  theta(rad) : Inport  Port=2  Unit=rad
  i(A) : Inport  Port=3  Unit=A
  MfIf : Inport  Port=4  Unit=V*s/rad
  Add{,1..3} (4 alike) : Sum
  Constant1 : Constant  Value=2*pi/3
  Constant2 : Constant  Value=2*pi/3
  Constant3 : Constant  Value=-2*pi/3
  Constant4 : Constant  Value=-2*pi/3
  Cos3 : Trigonometry  Operator=cos
  Cos4 : Trigonometry  Operator=cos
  Cos5 : Trigonometry  Operator=cos
  Dot Product : DotProduct  OutDataTypeStr=Inherit: Inherit via internal rule
  Dot Product1 : DotProduct  OutDataTypeStr=Inherit: Inherit via internal rule
  Gain1 : Gain  Gain=-1
  Multiply1 : Product
  Multiply2 : Product  Inputs=3
  Multiply3 : Product  Inputs=3
  Sin : Trigonometry
  Sin1 : Trigonometry
  Sin2 : Trigonometry
  Vector Concatenate : Concatenate  NumInputs=3
  Vector Concatenate1 : Concatenate  NumInputs=3
  Te(Nm) : Outport  Unit=N*m  VectorParamsAs1DForOutWhenUnconnected=off
  Q(Var) : Outport  Port=2  Unit=W  VectorParamsAs1DForOutWhenUnconnected=off
  e(V) : Outport  Port=3  Unit=V  VectorParamsAs1DForOutWhenUnconnected=off
  wires:
  Multiply3/1 -> Gain1/1
  Multiply1/1 -> Te(Nm)/1
  Constant2/1 -> Add/2
  Constant3/1 -> Add1/2
  Gain1/1 -> Q(Var)/1
  i(A)/1 -> [i]
  MfIf/1 -> [MfIf]
  theta(rad)/1 -> [theta]
  W(rad/s)/1 -> [W]
  [theta] -> Sin/1
  [MfIf] -> Multiply1/1
  [W] -> Multiply2/2
  [MfIf] -> Multiply2/3
  Multiply2/1 -> e(V)/1
  [theta] -> Add/1
  [theta] -> Add1/1
  Add/1 -> Sin1/1
  Add1/1 -> Sin2/1
  [MfIf] -> Multiply3/2
  Sin2/1 -> Vector Concatenate/2
  Sin/1 -> Vector Concatenate/1
  Sin1/1 -> Vector Concatenate/3
  Vector Concatenate/1 -> [SinH]
  [SinH] -> Multiply2/1
  [i] -> Dot Product/1
  [SinH] -> Dot Product/2
  Dot Product/1 -> Multiply1/2
  Cos5/1 -> Vector Concatenate1/2
  Vector Concatenate1/1 -> [CosH]
  Add2/1 -> Cos4/1
  Constant4/1 -> Add3/2
  Cos4/1 -> Vector Concatenate1/3
  Constant1/1 -> Add2/2
  [theta] -> Add2/1
  Add3/1 -> Cos5/1
  [theta] -> Add3/1
  Cos3/1 -> Vector Concatenate1/1
  [theta] -> Cos3/1
  [i] -> Dot Product1/1
  [CosH] -> Dot Product1/2
  [W] -> Multiply3/1
  Dot Product1/1 -> Multiply3/3
